simulink model "Controller"  (R2019a)
settings: Solver=VariableStepAuto  StartTime=0.0  StopTime=10.0  RelTol=1e-3
undefined symbols (not defined in the file): J, JD_0, Jw, r_ecef, t_orbit, v_ecef
libraries: sc_toolbox x6, vrlib x1
settings Model: Creator=mario  LastModifiedBy=mario
settings DataIOCC: ReturnWorkspaceOutputs=off
settings DebuggingCC: ArithmeticOperatorsInVariantConditions=warning

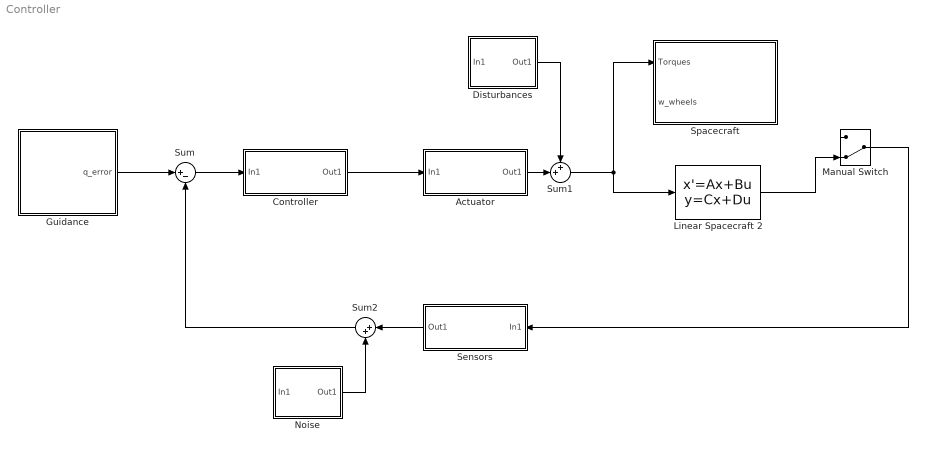
== system Controller ==
  Actuator : Subsystem
  Controller : Subsystem
  Disturbances : Subsystem
  Guidance : Subsystem
  "Linear Spacecraft 2 " : StateSpace  InitialCondition=0
  Manual Switch : ManualSwitch  CurrentSetting=0
  Noise : Subsystem
  Sensors : Subsystem
  Spacecraft : Subsystem
  Sum : Sum  Inputs=|+-
  Sum1 : Sum  Inputs=++|
  Sum2 : Sum  Inputs=|++
  wires:
  Controller/1(Out1) -> Actuator/1(In1)
  Sum1/1 -> Spacecraft/1(Torques), "Linear Spacecraft 2 "/1
  ? -> Manual Switch/1
  "Linear Spacecraft 2 "/1 -> Manual Switch/2
  Manual Switch/1 -> Sensors/1(In1)
  Sum/1 -> Controller/1(In1)
  Sum2/1 -> Sum/2
  Guidance/1(q_error) -> Sum/1
  Actuator/1(Out1) -> Sum1/2
  Disturbances/1(Out1) -> Sum1/1
  Noise/1(Out1) -> Sum2/2
  Sensors/1(Out1) -> Sum2/1

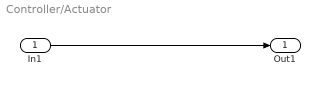
== system Controller/Actuator ==
  In1 : Inport
  Out1 : Outport
  wires:
  In1/1 -> Out1/1

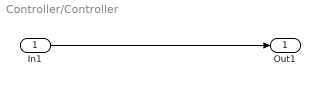
== system Controller/Controller ==
  In1 : Inport
  Out1 : Outport
  wires:
  In1/1 -> Out1/1

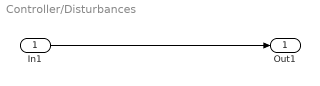
== system Controller/Disturbances ==
  In1 : Inport
  Out1 : Outport
  wires:
  In1/1 -> Out1/1

== system Controller/Guidance ==
  q_error : Outport

== system Controller/Noise ==
  In1 : Inport
  Out1 : Outport
  wires:
  In1/1 -> Out1/1

== system Controller/Sensors ==
  In1 : Inport
  Out1 : Outport
  wires:
  In1/1 -> Out1/1

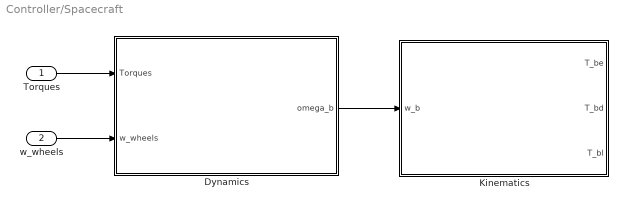
== system Controller/Spacecraft ==
  Torques : Inport
  w_wheels : Inport  Port=2
  Dynamics : Subsystem
  Kinematics : Subsystem
  wires:
  Torques/1 -> Dynamics/1(Torques)
  w_wheels/1 -> Dynamics/2(w_wheels)
  Dynamics/1(omega_b) -> Kinematics/1(w_b)

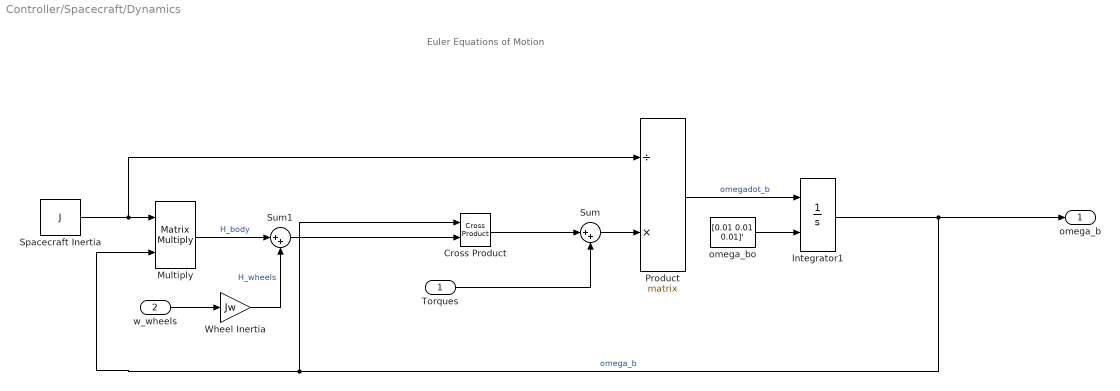
== system Controller/Spacecraft/Dynamics ==
  note: Euler Equations of Motion
  Torques : Inport
  w_wheels : Inport  Port=2
  Cross Product : vrlib/Utilities/Cross Product
      settings: SourceProductName=Simulink
  Integrator1 : Integrator  InitialConditionSource=external
  Multiply : Product  Multiplication=Matrix(*)
  Product : Product  Inputs=/*  Multiplication=Matrix(*)
  Spacecraft Inertia : Constant  Value=J
  Sum : Sum  Inputs=|++
  Sum1 : Sum  Inputs=|++
  Wheel Inertia : Gain  Gain=Jw
  omega_bo : Constant  Value=[0.01 0.01 0.01]'
  omega_b : Outport
  wires:
  Sum1/1 -> Cross Product/2
  Integrator1/1 -> Cross Product/1, Multiply/2, omega_b/1  "omega_b"
  Torques/1 -> Sum/2
  Cross Product/1 -> Sum/1
  Wheel Inertia/1 -> Sum1/2  "H_wheels"
  Spacecraft Inertia/1 -> Product/1, Multiply/1
  Sum/1 -> Product/2
  w_wheels/1 -> Wheel Inertia/1
  Product/1 -> Integrator1/1  "omegadot_b"
  Multiply/1 -> Sum1/1  "H_body"
  omega_bo/1 -> Integrator1/2

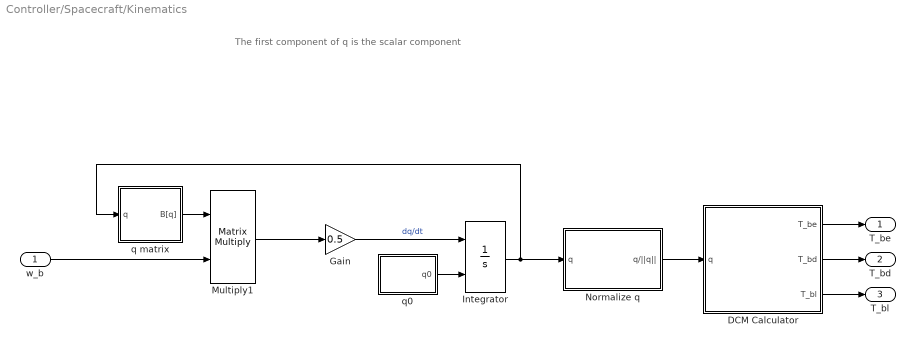
== system Controller/Spacecraft/Kinematics ==
  note: The first component of q is the scalar component
  w_b : Inport
  DCM Calculator : Subsystem
  Gain : Gain  Gain=0.5
  Integrator : Integrator  InitialConditionSource=external
  Multiply1 : Product  Multiplication=Matrix(*)
  Normalize q : Subsystem
  q matrix : Subsystem
  q0 : Subsystem
  T_be : Outport
  T_bd : Outport  Port=2
  T_bl : Outport  Port=3
  wires:
  Multiply1/1 -> Gain/1
  q matrix/1(B[q]) -> Multiply1/1
  q0/1(q0) -> Integrator/2
  Gain/1 -> Integrator/1  "dq/dt"
  Normalize q/1(q/||q||) -> DCM Calculator/1("q ")
  Integrator/1 -> Normalize q/1(q), q matrix/1(q)
  w_b/1 -> Multiply1/2
  DCM Calculator/1(T_be) -> T_be/1
  DCM Calculator/2(T_bd) -> T_bd/1
  DCM Calculator/3(T_bl) -> T_bl/1

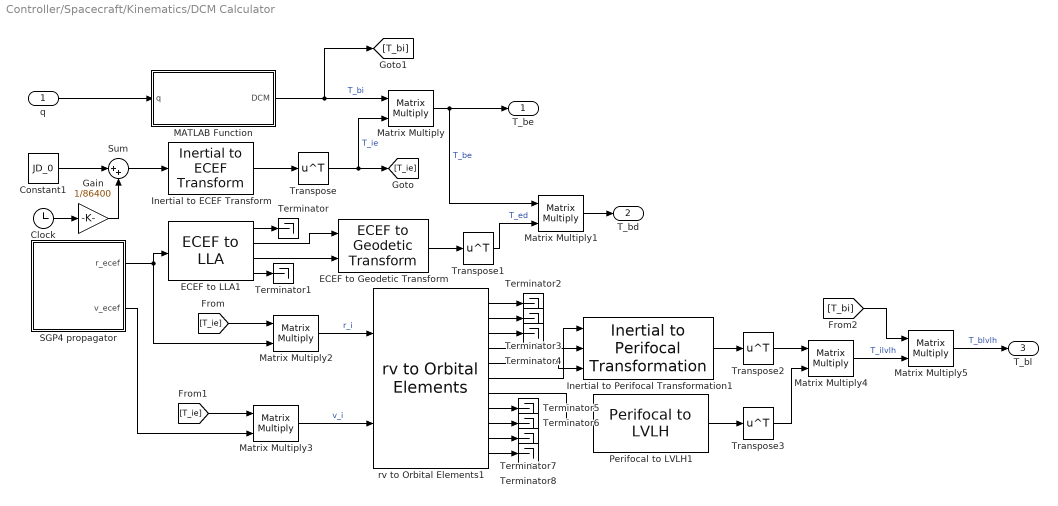
== system Controller/Spacecraft/Kinematics/DCM Calculator ==
  "q " : Inport
  Clock : Clock
  Constant1 : Constant  Value=JD_0
  ECEF to Geodetic Transform : sc_toolbox/Coordinates Transformations/ECEF to Geodetic Transform  SystemSampleTime=-1
      settings: SourceProductName=Spacecraft Toolbox
  ECEF to LLA1 : sc_toolbox/Coordinates Transformations/ECEF to LLA  SystemSampleTime=-1
      settings: SourceProductName=Spacecraft Toolbox
  Gain : Gain  Gain=1/86400
  Inertial to ECEF Transform : sc_toolbox/Coordinates Transformations/Inertial to ECEF Transform  SystemSampleTime=-1
      settings: SourceProductName=Spacecraft Toolbox
  Inertial to Perifocal Transformation1 : sc_toolbox/Coordinates Transformations/Inertial to Perifocal Transformation  SystemSampleTime=-1
      settings: SourceProductName=Spacecraft Toolbox
  MATLAB Function : MATLAB Function  TreatAsAtomicUnit=on
  Matrix Multiply{,1..5} (6 alike) : Product  Multiplication=Matrix(*)
  Perifocal to LVLH1 : sc_toolbox/Coordinates Transformations/Perifocal to LVLH  SystemSampleTime=-1
      settings: SourceProductName=Spacecraft Toolbox
  SGP4 propagator : Subsystem
  Sum : Sum  Inputs=|++
  Terminator{,1..8} (9 alike) : Terminator
  Transpose{,1..3} (4 alike) : Math  Operator=transpose  SaturateOnIntegerOverflow=on
  rv to Orbital Elements1 : sc_toolbox/Coordinates Transformations/rv to Orbital Elements  SystemSampleTime=-1
      settings: SourceProductName=Spacecraft Toolbox
  T_be : Outport
  T_bd : Outport  Port=2
  T_bl : Outport  Port=3
  wires:
  "q "/1 -> MATLAB Function/1(q)
  Gain/1 -> Sum/2
  Constant1/1 -> Sum/1
  Clock/1 -> Gain/1
  MATLAB Function/1(DCM) -> Matrix Multiply/1, [T_bi]  "T_bi"
  Sum/1 -> Inertial to ECEF Transform/1
  Inertial to ECEF Transform/1 -> Transpose/1
  Transpose/1 -> Matrix Multiply/2, [T_ie]  "T_ie"
  Matrix Multiply/1 -> Matrix Multiply1/1, T_be/1  "T_be"
  ECEF to LLA1/2 -> ECEF to Geodetic Transform/1
  ECEF to LLA1/3 -> ECEF to Geodetic Transform/2
  ECEF to LLA1/1 -> Terminator/1
  ECEF to LLA1/4 -> Terminator1/1
  ECEF to Geodetic Transform/1 -> Transpose1/1
  Transpose1/1 -> Matrix Multiply1/2  "T_ed"
  Matrix Multiply1/1 -> T_bd/1
  SGP4 propagator/1(r_ecef) -> ECEF to LLA1/1, Matrix Multiply2/2
  rv to Orbital Elements1/4 -> Inertial to Perifocal Transformation1/2
  rv to Orbital Elements1/5 -> Inertial to Perifocal Transformation1/3
  rv to Orbital Elements1/6 -> Inertial to Perifocal Transformation1/1
  Matrix Multiply2/1 -> rv to Orbital Elements1/1  "r_i"
  [T_ie] -> Matrix Multiply2/1
  [T_ie] -> Matrix Multiply3/1
  Matrix Multiply3/1 -> rv to Orbital Elements1/2  "v_i"
  SGP4 propagator/2(v_ecef) -> Matrix Multiply3/2
  rv to Orbital Elements1/7 -> Perifocal to LVLH1/1
  Inertial to Perifocal Transformation1/1 -> Transpose2/1
  Perifocal to LVLH1/1 -> Transpose3/1
  Transpose2/1 -> Matrix Multiply4/1
  Transpose3/1 -> Matrix Multiply4/2
  Matrix Multiply4/1 -> Matrix Multiply5/2  "T_ilvlh"
  [T_bi] -> Matrix Multiply5/1
  Matrix Multiply5/1 -> T_bl/1  "T_blvlh"
  rv to Orbital Elements1/1 -> Terminator2/1
  rv to Orbital Elements1/2 -> Terminator3/1
  rv to Orbital Elements1/3 -> Terminator4/1
  rv to Orbital Elements1/8 -> Terminator5/1
  rv to Orbital Elements1/9 -> Terminator6/1
  rv to Orbital Elements1/10 -> Terminator7/1
  rv to Orbital Elements1/11 -> Terminator8/1

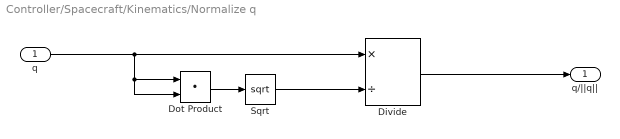
== system Controller/Spacecraft/Kinematics/Normalize q ==
  q : Inport
  Divide : Product  Inputs=*/
  Dot Product : DotProduct  InputSameDT=on  OutDataTypeStr=Inherit: Inherit via internal rule
  Sqrt : Sqrt  SaturateOnIntegerOverflow=on
  q/||q|| : Outport
  wires:
  q/1 -> Divide/1, Dot Product/2, Dot Product/1
  Sqrt/1 -> Divide/2
  Dot Product/1 -> Sqrt/1
  Divide/1 -> q/||q||/1

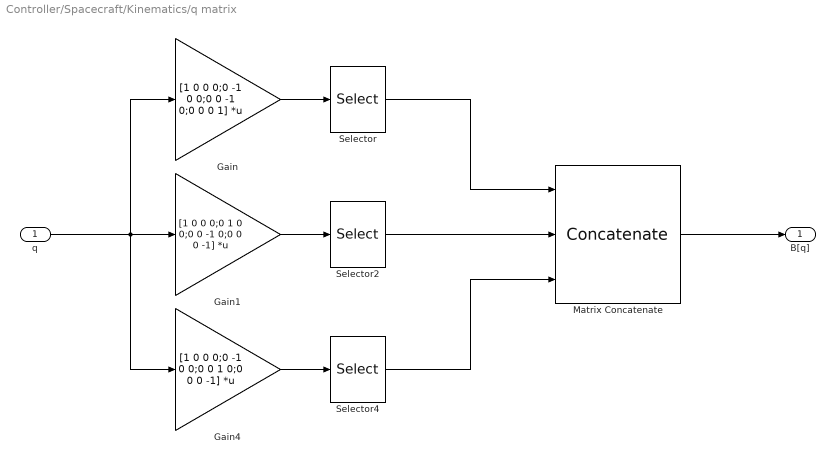
== system Controller/Spacecraft/Kinematics/q matrix ==
  q : Inport
  Gain : Gain  Gain=[1 0 0 0;0 -1 0 0;0 0 -1 0;0 0 0 1]  Multiplication=Matrix(K*u)
  Gain1 : Gain  Gain=[1 0 0 0;0 1 0 0;0 0 -1 0;0 0 0 -1]  Multiplication=Matrix(K*u)
  Gain4 : Gain  Gain=[1 0 0 0;0 -1 0 0;0 0 1 0;0 0 0 -1]  Multiplication=Matrix(K*u)
  Matrix Concatenate : Concatenate  NumInputs=3  Mode=Multidimensional array  ConcatenateDimension=2
  Selector : Selector  InputPortWidth=4  IndexOptions=Index vector (dialog)  Indices=[2 1 4 3]  OutputSizes=1
  Selector2 : Selector  InputPortWidth=4  IndexOptions=Index vector (dialog)  Indices=[3 4 1 2]  OutputSizes=1
  Selector4 : Selector  InputPortWidth=4  IndexOptions=Index vector (dialog)  Indices=[4 3 2 1]  OutputSizes=1
  B[q] : Outport
  wires:
  Gain4/1 -> Selector4/1
  Selector2/1 -> Matrix Concatenate/2
  Matrix Concatenate/1 -> B[q]/1
  Selector4/1 -> Matrix Concatenate/3
  q/1 -> Gain4/1, Gain/1, Gain1/1
  Selector/1 -> Matrix Concatenate/1
  Gain1/1 -> Selector2/1
  Gain/1 -> Selector/1

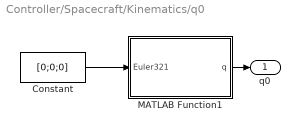
== system Controller/Spacecraft/Kinematics/q0 ==
  Constant : Constant  Value=[0;0;0]
  MATLAB Function1 : MATLAB Function  TreatAsAtomicUnit=on
  q0 : Outport
  wires:
  Constant/1 -> MATLAB Function1/1(Euler321)
  MATLAB Function1/1(q) -> q0/1

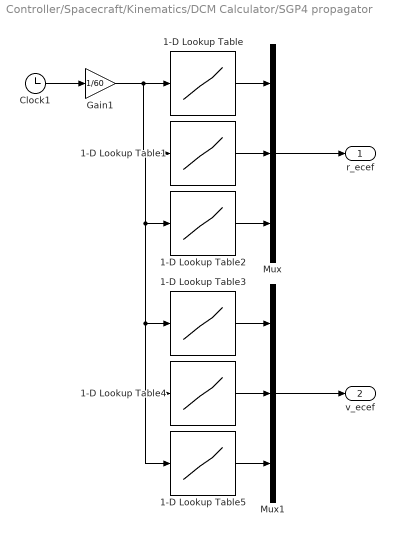
== system Controller/Spacecraft/Kinematics/DCM Calculator/SGP4 propagator ==
  1-D Lookup Table : Lookup_n-D  NumberOfTableDimensions=1  BreakpointsForDimension1=t_orbit  BreakpointsForDimension2=t_orbit  BreakpointsForDimension3=t_orbit  Table=r_ecef(:,1)  InternalRulePriority=Speed  RndMeth=Simplest  InputSameDT=on
  1-D Lookup Table1 : Lookup_n-D  NumberOfTableDimensions=1  BreakpointsForDimension1=t_orbit  BreakpointsForDimension2=t_orbit  BreakpointsForDimension3=t_orbit  Table=r_ecef(:,2)  InternalRulePriority=Speed  RndMeth=Simplest  InputSameDT=on
  1-D Lookup Table2 : Lookup_n-D  NumberOfTableDimensions=1  BreakpointsForDimension1=t_orbit  BreakpointsForDimension2=t_orbit  BreakpointsForDimension3=t_orbit  Table=r_ecef(:,3)  InternalRulePriority=Speed  RndMeth=Simplest  InputSameDT=on
  1-D Lookup Table3 : Lookup_n-D  NumberOfTableDimensions=1  BreakpointsForDimension1=t_orbit  BreakpointsForDimension2=t_orbit  BreakpointsForDimension3=t_orbit  Table=v_ecef(:,1)  InternalRulePriority=Speed  RndMeth=Simplest  InputSameDT=on
  1-D Lookup Table4 : Lookup_n-D  NumberOfTableDimensions=1  BreakpointsForDimension1=t_orbit  BreakpointsForDimension2=t_orbit  BreakpointsForDimension3=t_orbit  Table=v_ecef(:,2)  InternalRulePriority=Speed  RndMeth=Simplest  InputSameDT=on
  1-D Lookup Table5 : Lookup_n-D  NumberOfTableDimensions=1  BreakpointsForDimension1=t_orbit  BreakpointsForDimension2=t_orbit  BreakpointsForDimension3=t_orbit  Table=v_ecef(:,3)  InternalRulePriority=Speed  RndMeth=Simplest  InputSameDT=on
  Clock1 : Clock
  Gain1 : Gain  Gain=1/60
  Mux : Mux  Inputs=3
  Mux1 : Mux  Inputs=3
  r_ecef : Outport  VectorParamsAs1DForOutWhenUnconnected=on
  v_ecef : Outport  Port=2
  wires:
  1-D Lookup Table2/1 -> Mux/3
  Gain1/1 -> 1-D Lookup Table5/1, 1-D Lookup Table4/1, 1-D Lookup Table3/1, 1-D Lookup Table2/1, 1-D Lookup Table1/1, 1-D Lookup Table/1
  Clock1/1 -> Gain1/1
  1-D Lookup Table1/1 -> Mux/2
  1-D Lookup Table/1 -> Mux/1
  Mux/1 -> r_ecef/1
  1-D Lookup Table3/1 -> Mux1/1
  1-D Lookup Table4/1 -> Mux1/2
  1-D Lookup Table5/1 -> Mux1/3
  Mux1/1 -> v_ecef/1

== matlab function Controller/Spacecraft/Kinematics/q0/MATLAB Function1 ==
  data: Euler321 input; q output
function q = euler3212q(Euler321)
euler = [deg2rad(Euler321(1));deg2rad(Euler321(2));deg2rad(Euler321(3))];

c1 = cos(euler(1)/2);
s1 = sin(euler(1)/2);
c2 = cos(euler(2)/2);
s2 = sin(euler(2)/2);
c3 = cos(euler(3)/2);
s3 = sin(euler(3)/2);

q = [c1*c2*c3+s1*s2*s3 ;
     s1*c2*c3-c1*s2*s3;
     c1*s2*c3+s1*c2*s3;
     c1*c2*s3-s1*s2*c3];

== matlab function Controller/Spacecraft/Kinematics/DCM Calculator/MATLAB Function ==
  data: q input; DCM output
function DCM = q2dcm(q)
q1 = q(1);
qbar = [q(2);q(3);q(4)];
qtilde = [0 -qbar(3) qbar(2);qbar(3) 0 -qbar(1);-qbar(2) qbar(1) 0];

DCM = 2*(qbar*qbar') + (q1^2-qbar'*qbar)*eye(3) - 2*q1*qtilde;
